simulink model "MicrogridControl"  (R2025b)
settings: Solver=VariableStepAuto  StartTime=0.0  StopTime=8  FixedStep=Ts  RelTol=1e-3
PreLoadFcn:
  | NormalOperation;
  | MicrogridControlParam;
undefined symbols (not defined in the file): base, bessModeInitial, bessSystem, bessVoltage, breakerStatus, DiscIntNeverNeededParam, ee_sli_rtmsupport, event, gcbh, generator, gflInverter, gfmInverter, Inertia, lineInductance, lineResistance, machine, plannedIsland, pmsm, powerLimit, powerQuality, PV, PVInverter, ref, resync, solar, solarInsolationChange, systemFrequency, Ts, windController, windSystem, windTurbine
libraries: nesl_utility x234, ee_lib x174, fl_lib x143, eeGeneralControl x137, simulink x78, eeTransforms x47, slpidlib x23, nesl_utility_internal x12, eePwmGenerator x9, eeSinusoidalMeasurementV2 x9, custom_lib x7, batteryecm_lib x6
(part 13 of 25)

== system MicrogridControl/BESS/BESS Integrated1/Detailed/BESS Plant/Converter ==
  mabc : Inport
  Average : Subsystem  VariantControl=Average
  Switching : Subsystem  VariantControl=Switching
  + : PMIOPort  Side=Left
  - : PMIOPort  Port=2  Side=Left
  ~ : PMIOPort  Port=3  Side=Right

== system MicrogridControl/BESS/BESS Integrated1/Detailed/Filter & Measurements/PLL & Measurements ==
  V : Inport
  I : Inport  Port=2
  Measurement1 : Subsystem
  Measurement2 : Subsystem
  Subsystem : Subsystem
  Out Bus Element : Outport  PortName=VIbus  Element=Vq
  Out Bus Element1 : Outport  PortName=VIbus  Element=Vd
  Out Bus Element2 : Outport  PortName=VIbus  Element=Freq
  Out Bus Element3 : Outport  PortName=VIbus  Element=Theta
  Out Bus Element4 : Outport  PortName=VIbus  Element=Vmag
  Out Bus Element5 : Outport  PortName=VIbus  Element=Iq
  Out Bus Element6 : Outport  PortName=VIbus  Element=Id
  Out Bus Element7 : Outport  PortName=VIbus  Element=Iabc
  Out Bus Element8 : Outport  PortName=VIbus  Element=Vabc
  wires:
  Subsystem/6(Id1) -> Out Bus Element6/1
  Subsystem/7(Iq1) -> Out Bus Element5/1
  Measurement1/1(Vg) -> Subsystem/2(Iabc), Out Bus Element7/1
  I/1 -> Measurement1/1(u)
  Subsystem/1(mag) -> Out Bus Element4/1
  Measurement2/1(Vg) -> Subsystem/1(Vabc), Out Bus Element8/1
  Subsystem/4(Vd) -> Out Bus Element1/1
  Subsystem/3(angle) -> Out Bus Element3/1
  Subsystem/5(Vq) -> Out Bus Element/1
  Subsystem/2(freq) -> Out Bus Element2/1
  V/1 -> Measurement2/1(u)

== system MicrogridControl/BESS/BESS Integrated1/Simplified/Grid Following/Measurements ==
  Current and Voltage Sensor (Three-Phase)5 : ee_lib/Sensors & Transducers/Current and Voltage Sensor (Three-Phase)  vMeasurementType=ee.enum.vmeasurement.lg  outputUnit=ee.enum.unit.pu  SRated=plantRating*1000 A*V  VRated=Vac V  I_specify=off  I_priority=None  I=[0, 0, 0] A  I_nominal_specify=off  I_nominal_value=1  I_nominal_unit=A  V_specify=off  V_priority=None  V=[0, 0, 0] V  V_nominal_specify=off  V_nominal_value=1  V_nominal_unit=V
      settings: InternalSimscapePortConfiguration="{\"Bottom\":[],\"Left\":[{\"id\":\"N1\",\"label\":\"~1\",\"type\":\"foundation.electrical.three_phase\"}],\"Right\":[{\"id\":\"V_output\",\"label\":\"V\",\"type\":\"output\"},{\"id\":\"I_output\",\"label\":\"I\",\"type\":\"output\"},{\"id\":\"N2\",\"label\":\"~2\",\"type\":\"foundation.electrical.three_phase\"}],\"Top\":[]}"
  Gain1 : Gain  Gain=1/(plantRating*1000)
  Gain2 : Gain  Gain=1/(plantRating*1000)
  Low-Pass Filter (Discrete or Continuous)1 : eeGeneralControl/Low-Pass Filter (Discrete or Continuous)  K=1  T=0.1  B=inf  A=-inf  init_option=Inherited from block input  x0=0  Ts=-1
  Low-Pass Filter (Discrete or Continuous)2 : eeGeneralControl/Low-Pass Filter (Discrete or Continuous)  K=1  T=0.1  B=inf  A=-inf  init_option=Inherited from block input  x0=0  Ts=-1
  PS-Simulink Converter{,1..3} (4 alike) : nesl_utility/PS-Simulink Converter  PhysicalDomain=network_engine_domain  SubClassName=ps_output  LeftPortType=input  RightPortType=output  PseudoPeriodic=off  Frequencies=[]  VectorFormat=inherit  Unit=inherit  AffineConversion=off
  Power Sensor (Three-Phase) : ee_lib/Sensors & Transducers/Power Sensor (Three-Phase)  load_type=ee.enum.passive.type_balanced.balanced  f0=60 Hz
      settings: InternalSimscapePortConfiguration="{\"Bottom\":[],\"Left\":[{\"id\":\"N1\",\"label\":\"~1\",\"type\":\"foundation.electrical.three_phase\"}],\"Right\":[{\"id\":\"N2\",\"label\":\"~2\",\"type\":\"foundation.electrical.three_phase\"}],\"Top\":[{\"id\":\"Pm\",\"label\":\"P\",\"type\":\"output\"},{\"id\":\"Qm\",\"label\":\"Q\",\"type\":\"output\"}]}"
  In : PMIOPort  Side=Left
  ~ : PMIOPort  Port=2  Side=Right
  P : Outport
  Q : Outport  Port=2
  V : Outport  Port=3
  I : Outport  Port=4
  wires:
  Gain2/1 -> Q/1
  Gain1/1 -> P/1
  PS-Simulink Converter3/1 -> I/1
  PS-Simulink Converter2/1 -> V/1
  Low-Pass Filter (Discrete or Continuous)2/1 -> Gain2/1
  Low-Pass Filter (Discrete or Continuous)1/1 -> Gain1/1
  PS-Simulink Converter1/1 -> Low-Pass Filter (Discrete or Continuous)2/1
  PS-Simulink Converter/1 -> Low-Pass Filter (Discrete or Continuous)1/1
  connections:
  PS-Simulink Converter3/LConn1 -- Current and Voltage Sensor (Three-Phase)5/RConn2
  Power Sensor (Three-Phase)/RConn1 -- Current and Voltage Sensor (Three-Phase)5/LConn1
  PS-Simulink Converter1/LConn1 -- Power Sensor (Three-Phase)/LConn3
  ~/RConn1 -- Current and Voltage Sensor (Three-Phase)5/RConn3
  In/RConn1 -- Power Sensor (Three-Phase)/LConn1
  PS-Simulink Converter/LConn1 -- Power Sensor (Three-Phase)/LConn2
  PS-Simulink Converter2/LConn1 -- Current and Voltage Sensor (Three-Phase)5/RConn1

== system MicrogridControl/BESS/BESS Integrated1/Simplified/Grid Following/Power Limiter ==
  P : Inport
  SOC : Inport  Port=2
  V : Inport  Port=3
  Add : Sum
  Compare To Constant : simulink/Logic and Bit Operations/Compare To Constant  relop=<=  const=minSOC  OutDataTypeStr=boolean
  Compare To Constant1 : simulink/Logic and Bit Operations/Compare To Constant  relop=>=  const=maxSOC  OutDataTypeStr=boolean
  Constant : Constant  Value=maxSOC
  Constant1 : Constant  Value=0
  Constant2 : Constant  Value=minSOC
  Constant3 : Constant  Value=0
  Constant5 : Constant  Value=minSOC
  Data Type Conversion : DataTypeConversion  OutDataTypeStr=double  SaturateOnIntegerOverflow=off  RndMeth=Floor
  Delay1 : Delay  DelayLength=1
  Divide : Product  Inputs=*/
  Gain : Gain  Gain=-1/(Inf)
  GreaterThan : RelationalOperator  Operator=>  OutDataTypeStr=boolean  RndMeth=Simplest  InputSameDT=off
  GreaterThan1 : RelationalOperator  Operator=<  OutDataTypeStr=boolean  RndMeth=Simplest  InputSameDT=off
  GreaterThan3 : RelationalOperator  Operator=<  OutDataTypeStr=boolean  RndMeth=Simplest  InputSameDT=off
  NOR : Logic  Operator=NOR  IconShape=distinctive  AllPortsSameDT=off  OutDataTypeStr=boolean
  Product : Product
  Scope1 : Scope  NumInputPorts=2
  Scope2 : Scope
  Scope3 : Scope  NumInputPorts=3
  Switch : Switch  Criteria=u2 > Threshold  SaturateOnIntegerOverflow=off  InputSameDT=off
  Switch1 : Switch  Criteria=u2 > Threshold  SaturateOnIntegerOverflow=off  InputSameDT=off
  Switch2 : Switch  Criteria=u2 > Threshold  SaturateOnIntegerOverflow=off  InputSameDT=off
  POut : Outport
  SOCFlag : Outport  Port=2
  wires:
  Product/1 -> POut/1
  Gain/1 -> Add/1
  Data Type Conversion/1 -> Product/2
  NOR/1 -> Data Type Conversion/1
  Compare To Constant1/1 -> NOR/2
  Compare To Constant/1 -> NOR/1
  Add/1 -> Compare To Constant1/1, Compare To Constant/1
  Switch2/1 -> Product/1, Divide/1
  Switch/1 -> Switch2/3, Scope3/3
  SOC/1 -> GreaterThan/1, GreaterThan1/1, Scope2/1, GreaterThan3/1, Add/2
  Divide/1 -> Gain/1
  Delay1/1 -> Divide/2
  V/1 -> Delay1/1
  GreaterThan3/1 -> SOCFlag/1
  Constant5/1 -> GreaterThan3/2
  Constant/1 -> GreaterThan/2
  GreaterThan/1 -> Switch/2
  Constant1/1 -> Switch/1
  Constant2/1 -> GreaterThan1/2
  GreaterThan1/1 -> Switch1/2, Scope1/1
  Constant3/1 -> Switch1/1
  Switch1/1 -> Switch2/1, Scope3/1
  P/1 -> Switch/3, Switch1/3, Switch2/2, Scope3/2

== system MicrogridControl/BESS/BESS Integrated1/Simplified/Grid Following/SOC Estimation ==
  I : Inport
  Constant : Constant  Value=0.95
  Gain : Gain  Gain=-1/(100000)
  Integrator (Discrete or Continuous) : eeGeneralControl/Integrator (Discrete or Continuous)  LabelModeActiveChoice=Discrete  IntegratorMethod=Integration: Forward Euler  ExternalReset=level  LimitType=Anti-windup  B=inf  A=-inf  Ts=-1
  SOC : Outport
  wires:
  Integrator (Discrete or Continuous)/1 -> SOC/1
  Gain/1 -> Integrator (Discrete or Continuous)/1
  I/1 -> Gain/1
  Constant/1 -> Integrator (Discrete or Continuous)/3

== system MicrogridControl/BESS/BESS Integrated1/Simplified/Grid Forming/Limiter ==
  SOC : Inport
  Compare To Constant : simulink/Logic and Bit Operations/Compare To Constant  relop=<=  const=minSOC  OutDataTypeStr=boolean
  Compare To Constant1 : simulink/Logic and Bit Operations/Compare To Constant  relop=>=  const=maxSOC  OutDataTypeStr=boolean
  Data Type Conversion : DataTypeConversion  OutDataTypeStr=double  SaturateOnIntegerOverflow=off  RndMeth=Floor
  Delay : Delay  DelayLength=1  InputProcessing=Columns as channels (frame based)
  OR : Logic  Operator=OR  AllPortsSameDT=off  OutDataTypeStr=boolean
  Flag : Outport
  wires:
  Delay/1 -> Flag/1
  Data Type Conversion/1 -> Delay/1
  OR/1 -> Data Type Conversion/1
  Compare To Constant1/1 -> OR/2
  Compare To Constant/1 -> OR/1
  SOC/1 -> Compare To Constant1/1, Compare To Constant/1

== system MicrogridControl/BESS/BESS Integrated1/Simplified/Grid Forming/Measurements ==
  Current and Voltage Sensor (Three-Phase)5 : ee_lib/Sensors & Transducers/Current and Voltage Sensor (Three-Phase)  vMeasurementType=ee.enum.vmeasurement.lg  outputUnit=ee.enum.unit.pu  SRated=plantRating*1000 A*V  VRated=Vac V  I_specify=off  I_priority=None  I=[0, 0, 0] A  I_nominal_specify=off  I_nominal_value=1  I_nominal_unit=A  V_specify=off  V_priority=None  V=[0, 0, 0] V  V_nominal_specify=off  V_nominal_value=1  V_nominal_unit=V
      settings: InternalSimscapePortConfiguration="{\"Bottom\":[],\"Left\":[{\"id\":\"N1\",\"label\":\"~1\",\"type\":\"foundation.electrical.three_phase\"}],\"Right\":[{\"id\":\"V_output\",\"label\":\"V\",\"type\":\"output\"},{\"id\":\"I_output\",\"label\":\"I\",\"type\":\"output\"},{\"id\":\"N2\",\"label\":\"~2\",\"type\":\"foundation.electrical.three_phase\"}],\"Top\":[]}"
  Gain1 : Gain  Gain=1/(plantRating*1000)
  Gain2 : Gain  Gain=1/(plantRating*1000)
  PS-Simulink Converter{,1..3} (4 alike) : nesl_utility/PS-Simulink Converter  PhysicalDomain=network_engine_domain  SubClassName=ps_output  LeftPortType=input  RightPortType=output  PseudoPeriodic=off  Frequencies=[]  VectorFormat=inherit  Unit=inherit  AffineConversion=off
  Power Sensor (Three-Phase) : ee_lib/Sensors & Transducers/Power Sensor (Three-Phase)  load_type=ee.enum.passive.type_balanced.balanced  f0=60 Hz
      settings: InternalSimscapePortConfiguration="{\"Bottom\":[],\"Left\":[{\"id\":\"N1\",\"label\":\"~1\",\"type\":\"foundation.electrical.three_phase\"}],\"Right\":[{\"id\":\"N2\",\"label\":\"~2\",\"type\":\"foundation.electrical.three_phase\"}],\"Top\":[{\"id\":\"Pm\",\"label\":\"P\",\"type\":\"output\"},{\"id\":\"Qm\",\"label\":\"Q\",\"type\":\"output\"}]}"
  In : PMIOPort  Side=Left
  ~ : PMIOPort  Port=2  Side=Right
  P : Outport
  Q : Outport  Port=2
  V : Outport  Port=3
  I : Outport  Port=4
  wires:
  PS-Simulink Converter1/1 -> Gain2/1
  PS-Simulink Converter/1 -> Gain1/1
  PS-Simulink Converter2/1 -> V/1
  PS-Simulink Converter3/1 -> I/1
  Gain1/1 -> P/1
  Gain2/1 -> Q/1
  connections:
  PS-Simulink Converter2/LConn1 -- Current and Voltage Sensor (Three-Phase)5/RConn1
  PS-Simulink Converter/LConn1 -- Power Sensor (Three-Phase)/LConn2
  In/RConn1 -- Power Sensor (Three-Phase)/LConn1
  ~/RConn1 -- Current and Voltage Sensor (Three-Phase)5/RConn3
  PS-Simulink Converter1/LConn1 -- Power Sensor (Three-Phase)/LConn3
  Power Sensor (Three-Phase)/RConn1 -- Current and Voltage Sensor (Three-Phase)5/LConn1
  PS-Simulink Converter3/LConn1 -- Current and Voltage Sensor (Three-Phase)5/RConn2

== system MicrogridControl/BESS/BESS Integrated1/Simplified/Grid Forming/Reference Generator ==
  Mode : Inport
  PRef : Inport  Port=2
  P : Inport  Port=3
  QRef : Inport  Port=4
  Q : Inport  Port=5
  VRef : Inport  Port=6
  V : Inport  Port=7
  Gain : Gain  Gain=efficiency/100
  Gain2 : Gain  Gain=sqrt(3)/Vac
  If : If
  If Action Subsystem : Subsystem  TreatAsAtomicUnit=on
  If Action Subsystem1 : Subsystem  TreatAsAtomicUnit=on
  Merge : Merge
  Merge1 : Merge
  Vt : Outport
  Ph : Outport  Port=2
  wires:
  Gain/1 -> If Action Subsystem/1(PRef)
  Mode/1 -> If/1
  If/1 -> If Action Subsystem/Action
  PRef/1 -> Gain/1, If Action Subsystem1/1(PRef)
  QRef/1 -> If Action Subsystem/3(QRef)
  VRef/1 -> If Action Subsystem1/3(VRef)
  V/1 -> Gain2/1
  If/2 -> If Action Subsystem1/Action
  If Action Subsystem/1(Vt) -> Merge/1
  If Action Subsystem1/1(Vt) -> Merge/2
  If Action Subsystem/2(Ph) -> Merge1/1
  If Action Subsystem1/2(Ph) -> Merge1/2
  Merge1/1 -> Ph/1
  P/1 -> If Action Subsystem/2(P), If Action Subsystem1/2(P)
  Q/1 -> If Action Subsystem/4(Q)
  Gain2/1 -> If Action Subsystem1/4(V)
  Merge/1 -> Vt/1

== system MicrogridControl/BESS/BESS Integrated1/Simplified/Grid Forming/SOC Estimation ==
  P : Inport
  Constant : Constant  Value=Vdc
  Constant1 : Constant  Value=initialSOC
  Constant2 : Constant  Value=capacity
  Constant3 : Constant  Value=Inf
  Divide : Product  Inputs=*/
  Divide1 : Product  Inputs=*/
  Gain : Gain  Gain=-plantRating*1000
  Integrator (Discrete or Continuous) : eeGeneralControl/Integrator (Discrete or Continuous)  LabelModeActiveChoice=Discrete  IntegratorMethod=Integration: Forward Euler  ExternalReset=level  LimitType=Anti-windup  B=inf  A=-inf  Ts=-1
  String Compare : StringCompare
  String Constant : StringConstant  String=capacityType
  String Constant1 : StringConstant  String="\"Fixed\""
  Switch : Switch  Criteria=u2 > Threshold  SaturateOnIntegerOverflow=off  InputSameDT=off
  Meas : Outport
  wires:
  Gain/1 -> Divide/1
  P/1 -> Gain/1
  Constant/1 -> Divide/2
  Divide/1 -> Divide1/1
  Constant1/1 -> Integrator (Discrete or Continuous)/3
  Integrator (Discrete or Continuous)/1 -> Meas/1
  String Constant/1 -> String Compare/1
  String Constant1/1 -> String Compare/2
  String Compare/1 -> Switch/2
  Switch/1 -> Divide1/2
  Divide1/1 -> Integrator (Discrete or Continuous)/1
  Constant2/1 -> Switch/1
  Constant3/1 -> Switch/3

== system MicrogridControl/BESS/BESS Integrated3/Detailed/BESS Controller/Grid Following ==
  VRef : Inport
  FRef : Inport  Port=2
  PRef : Inport  Port=3
  QRef : Inport  Port=4
  Mode : Inport  Port=5
  Reset : Inport  Port=6
  In Bus Element3 : Inport  Port=7  PortName=VIBus  Element=Vd
  BusElementIn : Inport  Port=7  PortName=VIBus  Element=Vd
  In Bus Element2 : Inport  Port=7  PortName=VIBus  Element=Vq
  In Bus Element7 : Inport  Port=7  PortName=VIBus  Element=Theta
  BusElementIn1 : Inport  Port=7  PortName=VIBus  Element=Freq
  BusElementIn3 : Inport  Port=7  PortName=VIBus  Element=Id
  BusElementIn4 : Inport  Port=7  PortName=VIBus  Element=Iq
  Constant : Constant  Value=10
  Current_controller : Subsystem
  Inverse Park Transform1 : eeTransforms/Inverse Park Transform  AxisAlignment=Q-axis  PowerInvariant=off
  Reference Current : Subsystem
  Sum2 : Sum  Inputs=|+-
  Terminator : Terminator
  Terminator1 : Terminator
  Unit Delay : UnitDelay  SampleTime=Td  HasFrameUpgradeWarning=on
  Unit Delay1 : UnitDelay  SampleTime=Td  HasFrameUpgradeWarning=on
  Unit Delay2 : UnitDelay  SampleTime=Ts  HasFrameUpgradeWarning=on
  mabc : Outport
  wires:
  QRef/1 -> Reference Current/6(QRef)
  PRef/1 -> Reference Current/5(PRef)
  BusElementIn4/1 -> Current_controller/4(iq)
  BusElementIn3/1 -> Current_controller/2(ipvd)
  BusElementIn1/1 -> Unit Delay1/1
  BusElementIn/1 -> Unit Delay/1
  Unit Delay/1 -> Reference Current/2(V-mag)
  Unit Delay1/1 -> Sum2/2
  Reference Current/1(id_ref) -> Current_controller/1(id-ref)
  Reference Current/2(iq_ref) -> Current_controller/3(iqref)
  Sum2/1 -> Reference Current/3(del f)
  VRef/1 -> Reference Current/1(V_ref)
  FRef/1 -> Sum2/1
  In Bus Element7/1 -> Inverse Park Transform1/2
  In Bus Element3/1 -> Current_controller/5(Vd)
  Current_controller/1(mdq0) -> Inverse Park Transform1/1
  Unit Delay2/1 -> mabc/1
  Inverse Park Transform1/1 -> Unit Delay2/1
  In Bus Element2/1 -> Current_controller/6(Vq)
  Mode/1 -> Terminator/1
  Reset/1 -> Terminator1/1
  Constant/1 -> Reference Current/4(LVRT_iq)

== system MicrogridControl/BESS/BESS Integrated3/Detailed/BESS Controller/Grid Forming ==
  VRef : Inport
  FRef : Inport  Port=2
  PRef : Inport  Port=3
  QRef : Inport  Port=4
  Mode : Inport  Port=5
  Reset : Inport  Port=6
  Bus Element In : Inport  Port=7  PortName=VIBus  Element=Vabc
  BusElementIn : Inport  Port=7  PortName=VIBus  Element=Iabc
  Current Limiting : Subsystem
  Grid Voltage Reactive Power Support : Subsystem
  Measurement : Subsystem
      mask Display: image('meas2_1_7_7_2_2.png');
  Power Control : Subsystem
  Subsystem2 : Subsystem
      settings: PortSchema="{\"entries\":[{\"content\":{\"sides\":[{\"content\":{\"connectorIds\":[\"Out1\"]},\"type\":\"ConnectorPlacement.EquallySpacedRectSide\",\"uuid\":\"7526c1f7-0aba-4355-8bbd-47d168879ecb\"},{\"content\":{\"connectorIds\":[\"In1\",\"In2\"],\"side\":\"RIGHT\"},\"type\":\"ConnectorPlacement.EquallySpacedRectSide\",\"uuid\":\"1dda9693-ec76-4df0-8ad4-aaa83d2574b3\"},{\"content\":{\"side\":\"TOP\"},\"type\":\"ConnectorPlacement.EquallySpacedRectSide\",\"uuid\":\"71ea411b-eb5f-4279-ae23-08ebb3ff1ed6\"}]},\"type\":\"ConnectorPlacement.EquallySpacedConnector\",\"uuid\":\"19864e0c-0998-460d-9705-13c69283d4ec\"}],\"packageUris\":[\"http://schema.mathworks.com/mf0/Connector/R2020b\"],\"version\":\"1.0\"}"
  Terminator : Terminator
  Terminator1 : Terminator
  Terminator2 : Terminator
  VoltageCurrentControl : Subsystem
      settings: PortSchema="{\"entries\":[{\"content\":{\"sides\":[{\"content\":{\"connectorIds\":[\"In1\",\"In2\",\"In3\"]},\"type\":\"ConnectorPlacement.EquallySpacedRectSide\",\"uuid\":\"0bf15a12-7bc0-47e4-89bd-435769673763\"},{\"content\":{\"connectorIds\":[\"Out1\"],\"side\":\"RIGHT\"},\"type\":\"ConnectorPlacement.EquallySpacedRectSide\",\"uuid\":\"44a15d74-8878-4ec6-abe4-be0b1b609519\"},{\"content\":{\"connectorIds\":[\"In4\"],\"side\":\"TOP\"},\"type\":\"ConnectorPlacement.EquallySpacedRectSide\",\"uuid\":\"7a96781e-5638-4b2a-8101-d5785aae9f0f\"}]},\"type\":\"ConnectorPlacement.EquallySpacedConnector\",\"uuid\":\"4b3373ad-cf20-4175-894e-3bd1604dd0ce\"}],\"packageUris\":[\"http://schema.mathworks.com/mf0/Connector/R2020b\"],\"version\":\"1.0\"}"
  mabc : Outport
  wires:
  Reset/1 -> Subsystem2/2(Reset), VoltageCurrentControl/3(Reset)
  Mode/1 -> Power Control/6(CntrlFlag)
  VRef/1 -> Power Control/4(Vref)
  FRef/1 -> Power Control/5(Fref)
  Measurement/4(fmeas) -> Terminator2/1
  Grid Voltage Reactive Power Support/2(Qref) -> Power Control/3(Qref)
  Grid Voltage Reactive Power Support/1(Pref) -> Power Control/2(Pref)
  PRef/1 -> Grid Voltage Reactive Power Support/2(PrefInput)
  QRef/1 -> Grid Voltage Reactive Power Support/3(QrefInput)
  Current Limiting/1(currentLimiting) -> VoltageCurrentControl/1(currentLimiting)
  Power Control/2(activeControl) -> VoltageCurrentControl/2(activeControl)
  Power Control/1(reactiveControl) -> Current Limiting/2(reactiveControl)
  Power Control/3(angle) -> Measurement/3(Angle)
  Measurement/1(measure) -> Grid Voltage Reactive Power Support/1(measure), Power Control/1(measure), VoltageCurrentControl/4(measure), Current Limiting/1(measure)
  Measurement/3(Qmeas) -> Terminator1/1
  Measurement/2(Pmeas) -> Terminator/1
  BusElementIn/1 -> Measurement/2(Igabc)
  Bus Element In/1 -> Measurement/1(Vgabcc)
  VoltageCurrentControl/1(mabc) -> Subsystem2/1(In)
  Subsystem2/1(mabc) -> mabc/1

== system MicrogridControl/BESS/BESS Integrated3/Detailed/BESS Plant/Converter ==
  mabc : Inport
  Average : Subsystem  VariantControl=Average
  Switching : Subsystem  VariantControl=Switching
  + : PMIOPort  Side=Left
  - : PMIOPort  Port=2  Side=Left
  ~ : PMIOPort  Port=3  Side=Right

== system MicrogridControl/BESS/BESS Integrated3/Detailed/Filter & Measurements/PLL & Measurements ==
  V : Inport
  I : Inport  Port=2
  Measurement1 : Subsystem
  Measurement2 : Subsystem
  Subsystem : Subsystem
  Out Bus Element : Outport  PortName=VIbus  Element=Vq
  Out Bus Element1 : Outport  PortName=VIbus  Element=Vd
  Out Bus Element2 : Outport  PortName=VIbus  Element=Freq
  Out Bus Element3 : Outport  PortName=VIbus  Element=Theta
  Out Bus Element4 : Outport  PortName=VIbus  Element=Vmag
  Out Bus Element5 : Outport  PortName=VIbus  Element=Iq
  Out Bus Element6 : Outport  PortName=VIbus  Element=Id
  Out Bus Element7 : Outport  PortName=VIbus  Element=Iabc
  Out Bus Element8 : Outport  PortName=VIbus  Element=Vabc
  wires:
  Subsystem/6(Id1) -> Out Bus Element6/1
  Subsystem/7(Iq1) -> Out Bus Element5/1
  Measurement1/1(Vg) -> Subsystem/2(Iabc), Out Bus Element7/1
  I/1 -> Measurement1/1(u)
  Subsystem/1(mag) -> Out Bus Element4/1
  Measurement2/1(Vg) -> Subsystem/1(Vabc), Out Bus Element8/1
  Subsystem/4(Vd) -> Out Bus Element1/1
  Subsystem/3(angle) -> Out Bus Element3/1
  Subsystem/5(Vq) -> Out Bus Element/1
  Subsystem/2(freq) -> Out Bus Element2/1
  V/1 -> Measurement2/1(u)

== system MicrogridControl/BESS/BESS Integrated3/Simplified/Grid Following/Measurements ==
  Current and Voltage Sensor (Three-Phase)5 : ee_lib/Sensors & Transducers/Current and Voltage Sensor (Three-Phase)  vMeasurementType=ee.enum.vmeasurement.lg  outputUnit=ee.enum.unit.pu  SRated=plantRating*1000 A*V  VRated=Vac V  I_specify=off  I_priority=None  I=[0, 0, 0] A  I_nominal_specify=off  I_nominal_value=1  I_nominal_unit=A  V_specify=off  V_priority=None  V=[0, 0, 0] V  V_nominal_specify=off  V_nominal_value=1  V_nominal_unit=V
      settings: InternalSimscapePortConfiguration="{\"Bottom\":[],\"Left\":[{\"id\":\"N1\",\"label\":\"~1\",\"type\":\"foundation.electrical.three_phase\"}],\"Right\":[{\"id\":\"V_output\",\"label\":\"V\",\"type\":\"output\"},{\"id\":\"I_output\",\"label\":\"I\",\"type\":\"output\"},{\"id\":\"N2\",\"label\":\"~2\",\"type\":\"foundation.electrical.three_phase\"}],\"Top\":[]}"
  Gain1 : Gain  Gain=1/(plantRating*1000)
  Gain2 : Gain  Gain=1/(plantRating*1000)
  Low-Pass Filter (Discrete or Continuous)1 : eeGeneralControl/Low-Pass Filter (Discrete or Continuous)  K=1  T=0.1  B=inf  A=-inf  init_option=Inherited from block input  x0=0  Ts=-1
  Low-Pass Filter (Discrete or Continuous)2 : eeGeneralControl/Low-Pass Filter (Discrete or Continuous)  K=1  T=0.1  B=inf  A=-inf  init_option=Inherited from block input  x0=0  Ts=-1
  PS-Simulink Converter{,1..3} (4 alike) : nesl_utility/PS-Simulink Converter  PhysicalDomain=network_engine_domain  SubClassName=ps_output  LeftPortType=input  RightPortType=output  PseudoPeriodic=off  Frequencies=[]  VectorFormat=inherit  Unit=inherit  AffineConversion=off
  Power Sensor (Three-Phase) : ee_lib/Sensors & Transducers/Power Sensor (Three-Phase)  load_type=ee.enum.passive.type_balanced.balanced  f0=60 Hz
      settings: InternalSimscapePortConfiguration="{\"Bottom\":[],\"Left\":[{\"id\":\"N1\",\"label\":\"~1\",\"type\":\"foundation.electrical.three_phase\"}],\"Right\":[{\"id\":\"N2\",\"label\":\"~2\",\"type\":\"foundation.electrical.three_phase\"}],\"Top\":[{\"id\":\"Pm\",\"label\":\"P\",\"type\":\"output\"},{\"id\":\"Qm\",\"label\":\"Q\",\"type\":\"output\"}]}"
  In : PMIOPort  Side=Left
  ~ : PMIOPort  Port=2  Side=Right
  P : Outport
  Q : Outport  Port=2
  V : Outport  Port=3
  I : Outport  Port=4
  wires:
  Gain2/1 -> Q/1
  Gain1/1 -> P/1
  PS-Simulink Converter3/1 -> I/1
  PS-Simulink Converter2/1 -> V/1
  Low-Pass Filter (Discrete or Continuous)2/1 -> Gain2/1
  Low-Pass Filter (Discrete or Continuous)1/1 -> Gain1/1
  PS-Simulink Converter1/1 -> Low-Pass Filter (Discrete or Continuous)2/1
  PS-Simulink Converter/1 -> Low-Pass Filter (Discrete or Continuous)1/1
  connections:
  PS-Simulink Converter3/LConn1 -- Current and Voltage Sensor (Three-Phase)5/RConn2
  Power Sensor (Three-Phase)/RConn1 -- Current and Voltage Sensor (Three-Phase)5/LConn1
  PS-Simulink Converter1/LConn1 -- Power Sensor (Three-Phase)/LConn3
  ~/RConn1 -- Current and Voltage Sensor (Three-Phase)5/RConn3
  In/RConn1 -- Power Sensor (Three-Phase)/LConn1
  PS-Simulink Converter/LConn1 -- Power Sensor (Three-Phase)/LConn2
  PS-Simulink Converter2/LConn1 -- Current and Voltage Sensor (Three-Phase)5/RConn1

== system MicrogridControl/BESS/BESS Integrated3/Simplified/Grid Following/Power Limiter ==
  P : Inport
  SOC : Inport  Port=2
  V : Inport  Port=3
  Add : Sum
  Compare To Constant : simulink/Logic and Bit Operations/Compare To Constant  relop=<=  const=minSOC  OutDataTypeStr=boolean
  Compare To Constant1 : simulink/Logic and Bit Operations/Compare To Constant  relop=>=  const=maxSOC  OutDataTypeStr=boolean
  Constant : Constant  Value=maxSOC
  Constant1 : Constant  Value=0
  Constant2 : Constant  Value=minSOC
  Constant3 : Constant  Value=0
  Constant5 : Constant  Value=minSOC
  Data Type Conversion : DataTypeConversion  OutDataTypeStr=double  SaturateOnIntegerOverflow=off  RndMeth=Floor
  Delay1 : Delay  DelayLength=1
  Divide : Product  Inputs=*/
  Gain : Gain  Gain=-1/(Inf)
  GreaterThan : RelationalOperator  Operator=>  OutDataTypeStr=boolean  RndMeth=Simplest  InputSameDT=off
  GreaterThan1 : RelationalOperator  Operator=<  OutDataTypeStr=boolean  RndMeth=Simplest  InputSameDT=off
  GreaterThan3 : RelationalOperator  Operator=<  OutDataTypeStr=boolean  RndMeth=Simplest  InputSameDT=off
  NOR : Logic  Operator=NOR  IconShape=distinctive  AllPortsSameDT=off  OutDataTypeStr=boolean
  Product : Product
  Scope1 : Scope  NumInputPorts=2
  Scope2 : Scope
  Scope3 : Scope  NumInputPorts=3
  Switch : Switch  Criteria=u2 > Threshold  SaturateOnIntegerOverflow=off  InputSameDT=off
  Switch1 : Switch  Criteria=u2 > Threshold  SaturateOnIntegerOverflow=off  InputSameDT=off
  Switch2 : Switch  Criteria=u2 > Threshold  SaturateOnIntegerOverflow=off  InputSameDT=off
  POut : Outport
  SOCFlag : Outport  Port=2
  wires:
  Product/1 -> POut/1
  Gain/1 -> Add/1
  Data Type Conversion/1 -> Product/2
  NOR/1 -> Data Type Conversion/1
  Compare To Constant1/1 -> NOR/2
  Compare To Constant/1 -> NOR/1
  Add/1 -> Compare To Constant1/1, Compare To Constant/1
  Switch2/1 -> Product/1, Divide/1
  Switch/1 -> Switch2/3, Scope3/3
  SOC/1 -> GreaterThan/1, GreaterThan1/1, Scope2/1, GreaterThan3/1, Add/2
  Divide/1 -> Gain/1
  Delay1/1 -> Divide/2
  V/1 -> Delay1/1
  GreaterThan3/1 -> SOCFlag/1
  Constant5/1 -> GreaterThan3/2
  Constant/1 -> GreaterThan/2
  GreaterThan/1 -> Switch/2
  Constant1/1 -> Switch/1
  Constant2/1 -> GreaterThan1/2
  GreaterThan1/1 -> Switch1/2, Scope1/1
  Constant3/1 -> Switch1/1
  Switch1/1 -> Switch2/1, Scope3/1
  P/1 -> Switch/3, Switch1/3, Switch2/2, Scope3/2

== system MicrogridControl/BESS/BESS Integrated3/Simplified/Grid Following/SOC Estimation ==
  I : Inport
  Constant : Constant  Value=0.95
  Gain : Gain  Gain=-1/(100000)
  Integrator (Discrete or Continuous) : eeGeneralControl/Integrator (Discrete or Continuous)  LabelModeActiveChoice=Discrete  IntegratorMethod=Integration: Forward Euler  ExternalReset=level  LimitType=Anti-windup  B=inf  A=-inf  Ts=-1
  SOC : Outport
  wires:
  Integrator (Discrete or Continuous)/1 -> SOC/1
  Gain/1 -> Integrator (Discrete or Continuous)/1
  I/1 -> Gain/1
  Constant/1 -> Integrator (Discrete or Continuous)/3

== system MicrogridControl/BESS/BESS Integrated3/Simplified/Grid Forming/Limiter ==
  SOC : Inport
  Compare To Constant : simulink/Logic and Bit Operations/Compare To Constant  relop=<=  const=minSOC  OutDataTypeStr=boolean
  Compare To Constant1 : simulink/Logic and Bit Operations/Compare To Constant  relop=>=  const=maxSOC  OutDataTypeStr=boolean
  Data Type Conversion : DataTypeConversion  OutDataTypeStr=double  SaturateOnIntegerOverflow=off  RndMeth=Floor
  Delay : Delay  DelayLength=1  InputProcessing=Columns as channels (frame based)
  OR : Logic  Operator=OR  AllPortsSameDT=off  OutDataTypeStr=boolean
  Flag : Outport
  wires:
  Delay/1 -> Flag/1
  Data Type Conversion/1 -> Delay/1
  OR/1 -> Data Type Conversion/1
  Compare To Constant1/1 -> OR/2
  Compare To Constant/1 -> OR/1
  SOC/1 -> Compare To Constant1/1, Compare To Constant/1

== system MicrogridControl/BESS/BESS Integrated3/Simplified/Grid Forming/Measurements ==
  Current and Voltage Sensor (Three-Phase)5 : ee_lib/Sensors & Transducers/Current and Voltage Sensor (Three-Phase)  vMeasurementType=ee.enum.vmeasurement.lg  outputUnit=ee.enum.unit.pu  SRated=plantRating*1000 A*V  VRated=Vac V  I_specify=off  I_priority=None  I=[0, 0, 0] A  I_nominal_specify=off  I_nominal_value=1  I_nominal_unit=A  V_specify=off  V_priority=None  V=[0, 0, 0] V  V_nominal_specify=off  V_nominal_value=1  V_nominal_unit=V
      settings: InternalSimscapePortConfiguration="{\"Bottom\":[],\"Left\":[{\"id\":\"N1\",\"label\":\"~1\",\"type\":\"foundation.electrical.three_phase\"}],\"Right\":[{\"id\":\"V_output\",\"label\":\"V\",\"type\":\"output\"},{\"id\":\"I_output\",\"label\":\"I\",\"type\":\"output\"},{\"id\":\"N2\",\"label\":\"~2\",\"type\":\"foundation.electrical.three_phase\"}],\"Top\":[]}"
  Gain1 : Gain  Gain=1/(plantRating*1000)
  Gain2 : Gain  Gain=1/(plantRating*1000)
  PS-Simulink Converter{,1..3} (4 alike) : nesl_utility/PS-Simulink Converter  PhysicalDomain=network_engine_domain  SubClassName=ps_output  LeftPortType=input  RightPortType=output  PseudoPeriodic=off  Frequencies=[]  VectorFormat=inherit  Unit=inherit  AffineConversion=off
  Power Sensor (Three-Phase) : ee_lib/Sensors & Transducers/Power Sensor (Three-Phase)  load_type=ee.enum.passive.type_balanced.balanced  f0=60 Hz
      settings: InternalSimscapePortConfiguration="{\"Bottom\":[],\"Left\":[{\"id\":\"N1\",\"label\":\"~1\",\"type\":\"foundation.electrical.three_phase\"}],\"Right\":[{\"id\":\"N2\",\"label\":\"~2\",\"type\":\"foundation.electrical.three_phase\"}],\"Top\":[{\"id\":\"Pm\",\"label\":\"P\",\"type\":\"output\"},{\"id\":\"Qm\",\"label\":\"Q\",\"type\":\"output\"}]}"
  In : PMIOPort  Side=Left
  ~ : PMIOPort  Port=2  Side=Right
  P : Outport
  Q : Outport  Port=2
  V : Outport  Port=3
  I : Outport  Port=4
  wires:
  PS-Simulink Converter1/1 -> Gain2/1
  PS-Simulink Converter/1 -> Gain1/1
  PS-Simulink Converter2/1 -> V/1
  PS-Simulink Converter3/1 -> I/1
  Gain1/1 -> P/1
  Gain2/1 -> Q/1
  connections:
  PS-Simulink Converter2/LConn1 -- Current and Voltage Sensor (Three-Phase)5/RConn1
  PS-Simulink Converter/LConn1 -- Power Sensor (Three-Phase)/LConn2
  In/RConn1 -- Power Sensor (Three-Phase)/LConn1
  ~/RConn1 -- Current and Voltage Sensor (Three-Phase)5/RConn3
  PS-Simulink Converter1/LConn1 -- Power Sensor (Three-Phase)/LConn3
  Power Sensor (Three-Phase)/RConn1 -- Current and Voltage Sensor (Three-Phase)5/LConn1
  PS-Simulink Converter3/LConn1 -- Current and Voltage Sensor (Three-Phase)5/RConn2

== system MicrogridControl/BESS/BESS Integrated3/Simplified/Grid Forming/Reference Generator ==
  Mode : Inport
  PRef : Inport  Port=2
  P : Inport  Port=3
  QRef : Inport  Port=4
  Q : Inport  Port=5
  VRef : Inport  Port=6
  V : Inport  Port=7
  Gain : Gain  Gain=efficiency/100
  Gain2 : Gain  Gain=sqrt(3)/Vac
  If : If
  If Action Subsystem : Subsystem  TreatAsAtomicUnit=on
  If Action Subsystem1 : Subsystem  TreatAsAtomicUnit=on
  Merge : Merge
  Merge1 : Merge
  Vt : Outport
  Ph : Outport  Port=2
  wires:
  Gain/1 -> If Action Subsystem/1(PRef)
  Mode/1 -> If/1
  If/1 -> If Action Subsystem/Action
  PRef/1 -> Gain/1, If Action Subsystem1/1(PRef)
  QRef/1 -> If Action Subsystem/3(QRef)
  VRef/1 -> If Action Subsystem1/3(VRef)
  V/1 -> Gain2/1
  If/2 -> If Action Subsystem1/Action
  If Action Subsystem/1(Vt) -> Merge/1
  If Action Subsystem1/1(Vt) -> Merge/2
  If Action Subsystem/2(Ph) -> Merge1/1
  If Action Subsystem1/2(Ph) -> Merge1/2
  Merge1/1 -> Ph/1
  P/1 -> If Action Subsystem/2(P), If Action Subsystem1/2(P)
  Q/1 -> If Action Subsystem/4(Q)
  Gain2/1 -> If Action Subsystem1/4(V)
  Merge/1 -> Vt/1

== system MicrogridControl/BESS/BESS Integrated3/Simplified/Grid Forming/SOC Estimation ==
  P : Inport
  Constant : Constant  Value=Vdc
  Constant1 : Constant  Value=initialSOC
  Constant2 : Constant  Value=capacity
  Constant3 : Constant  Value=Inf
  Divide : Product  Inputs=*/
  Divide1 : Product  Inputs=*/
  Gain : Gain  Gain=-plantRating*1000
  Integrator (Discrete or Continuous) : eeGeneralControl/Integrator (Discrete or Continuous)  LabelModeActiveChoice=Discrete  IntegratorMethod=Integration: Forward Euler  ExternalReset=level  LimitType=Anti-windup  B=inf  A=-inf  Ts=-1
  String Compare : StringCompare
  String Constant : StringConstant  String=capacityType
  String Constant1 : StringConstant  String="\"Fixed\""
  Switch : Switch  Criteria=u2 > Threshold  SaturateOnIntegerOverflow=off  InputSameDT=off
  Meas : Outport
  wires:
  Gain/1 -> Divide/1
  P/1 -> Gain/1
  Constant/1 -> Divide/2
  Divide/1 -> Divide1/1
  Constant1/1 -> Integrator (Discrete or Continuous)/3
  Integrator (Discrete or Continuous)/1 -> Meas/1
  String Constant/1 -> String Compare/1
  String Constant1/1 -> String Compare/2
  String Compare/1 -> Switch/2
  Switch/1 -> Divide1/2
  Divide1/1 -> Integrator (Discrete or Continuous)/1
  Constant2/1 -> Switch/1
  Constant3/1 -> Switch/3

== system MicrogridControl/Generator/Generator Integrated/Detailed/Governor and Prime Mover /Governor ==
  pu_velocity : Inport
  PRef : Inport  Port=2
  1/T_G : Gain  Gain=1/T_G
  1/droop : Gain  Gain=1/(droop_percentage/100)
  Delta load setpoint : Sum  Inputs=+-|
  Delta speed : Sum  Inputs=-+|
  Discrete-Time Integrator1 : DiscreteIntegrator  InitialCondition=pu_torque0  SampleTime=-1  ICPrevOutput=DiscIntNeverNeededParam  ICPrevScaledInput=DiscIntNeverNeededParam
  Scope : Scope  NumInputPorts=2
  Scope1 : Scope  NumInputPorts=2
  Speed_ref : Constant  Value=pu_speed_reference
  Subtract : Sum  Inputs=|+-
  delta_y : Outport  VectorParamsAs1DForOutWhenUnconnected=off
  wires:
  PRef/1 -> Delta load setpoint/1
  Discrete-Time Integrator1/1 -> Subtract/2, delta_y/1, Scope1/2
  1/T_G/1 -> Discrete-Time Integrator1/1
  Subtract/1 -> 1/T_G/1, Scope1/1
  Delta load setpoint/1 -> Subtract/1
  1/droop/1 -> Delta load setpoint/2
  pu_velocity/1 -> Delta speed/2, Scope/2
  Delta speed/1 -> 1/droop/1, Scope/1
  Speed_ref/1 -> Delta speed/1

== system MicrogridControl/Generator/Generator Integrated/Detailed/Governor and Prime Mover /Non-reheat turbine ==
  delta_y : Inport
  1/T_CH : Gain  Gain=1/T_CH
  Discrete-Time Integrator1 : DiscreteIntegrator  InitialCondition=pu_torque0  SampleTime=-1  ICPrevOutput=DiscIntNeverNeededParam  ICPrevScaledInput=DiscIntNeverNeededParam
  Scope : Scope  NumInputPorts=2
  Sum : Sum  Inputs=|+-
  torque : Outport  VectorParamsAs1DForOutWhenUnconnected=off
  wires:
  Discrete-Time Integrator1/1 -> torque/1, Scope/1, Sum/2
  1/T_CH/1 -> Discrete-Time Integrator1/1
  Sum/1 -> 1/T_CH/1
  delta_y/1 -> Sum/1, Scope/2

== system MicrogridControl/Microgrid Controller/Microgrid Control Functions/Black Start/Voltage Reference/Voltage Level 1 ==
  Enable : Inport
  Constant : Constant
  Constant1 : Constant  Value=0
  Constant2 : Constant  DisableCoverage=on  Value=-(delayLevel1)  OutDataTypeStr=Inherit: Inherit via back propagation  SampleTime=Ts
  Discrete-Time Integrator : DiscreteIntegrator  SampleTime=Ts  OutDataTypeStr=double  ICPrevOutput=DiscIntNeverNeededParam  ICPrevScaledInput=DiscIntNeverNeededParam
  Output : Sum  Inputs=|++  InputSameDT=on  SaturateOnIntegerOverflow=on  OutDataTypeStr=Inherit: Same as first input
  Product : Product  DisableCoverage=on  InputSameDT=on  SaturateOnIntegerOverflow=on  OutDataTypeStr=Inherit: Same as first input
  Saturation : Saturate  UpperLimit=voltageLevel1  LowerLimit=0
  Step : Step  Commented=on  DisableCoverage=on  Time=controllerBlackStart+delayLevel1  OutDataTypeStr=fixdt('double', 'DataTypeOverride', 'Off')  SampleTime=Ts
  Level 1 : Outport
  wires:
  Constant1/1 -> Output/2
  Constant/1 -> Product/1
  Enable/1 -> Discrete-Time Integrator/1
  Output/1 -> Saturation/1
  Product/1 -> Output/1
  Saturation/1 -> Level 1/1
  Discrete-Time Integrator/1 -> Product/2

== system MicrogridControl/Microgrid Controller/Microgrid Control Functions/Black Start/Voltage Reference/Voltage Level 2 ==
  Enable : Inport
  Constant : Constant
  Constant1 : Constant  Value=0
  Constant2 : Constant  Commented=on  DisableCoverage=on  Value=-(delayLevel2)  OutDataTypeStr=Inherit: Inherit via back propagation  SampleTime=Ts
  Discrete-Time Integrator : DiscreteIntegrator  SampleTime=Ts  OutDataTypeStr=double  ICPrevOutput=DiscIntNeverNeededParam  ICPrevScaledInput=DiscIntNeverNeededParam
  Output : Sum  Inputs=|++  InputSameDT=on  SaturateOnIntegerOverflow=on  OutDataTypeStr=Inherit: Same as first input
  Product : Product  DisableCoverage=on  InputSameDT=on  SaturateOnIntegerOverflow=on  OutDataTypeStr=Inherit: Same as first input
  Saturation : Saturate  UpperLimit=voltageLevel2  LowerLimit=0
  Step : Step  Commented=on  DisableCoverage=on  Time=delayLevel1+delayLevel2  OutDataTypeStr=fixdt('double', 'DataTypeOverride', 'Off')  SampleTime=Ts
  Level 2 : Outport
  wires:
  Constant1/1 -> Output/2
  Constant/1 -> Product/1
  Enable/1 -> Discrete-Time Integrator/1
  Discrete-Time Integrator/1 -> Product/2
  Saturation/1 -> Level 2/1
  Product/1 -> Output/1
  Output/1 -> Saturation/1

== system MicrogridControl/Microgrid Controller/Microgrid Control Functions/Black Start/Voltage Reference/Voltage Level 3 ==
  Enable : Inport
  Constant : Constant
  Constant1 : Constant  Value=0
  Constant2 : Constant  Commented=on  DisableCoverage=on  Value=-(delayLevel3+delayLevel3)  OutDataTypeStr=Inherit: Inherit via back propagation  SampleTime=Ts
  Discrete-Time Integrator : DiscreteIntegrator  SampleTime=Ts  OutDataTypeStr=double  ICPrevOutput=DiscIntNeverNeededParam  ICPrevScaledInput=DiscIntNeverNeededParam
  Output : Sum  Inputs=|++  InputSameDT=on  SaturateOnIntegerOverflow=on  OutDataTypeStr=Inherit: Same as first input
  Product : Product  DisableCoverage=on  InputSameDT=on  SaturateOnIntegerOverflow=on  OutDataTypeStr=Inherit: Same as first input
  Saturation : Saturate  UpperLimit=voltageLevel3  LowerLimit=0
  Step : Step  Commented=on  DisableCoverage=on  Time=delayLevel1+delayLevel2+delayLevel3  OutDataTypeStr=fixdt('double', 'DataTypeOverride', 'Off')  SampleTime=Ts
  Level 3 : Outport
  wires:
  Constant1/1 -> Output/2
  Constant/1 -> Product/1
  Enable/1 -> Discrete-Time Integrator/1
  Output/1 -> Saturation/1
  Product/1 -> Output/1
  Saturation/1 -> Level 3/1
  Discrete-Time Integrator/1 -> Product/2

== system MicrogridControl/Microgrid Controller/Microgrid Control Functions/Resynchronization/Synch Voltage/Subsystem2 ==
  MicrogridController : Inport
  ControlRoom : Inport  Port=2
  Constant : Constant  Value=1.05
  Switch : Switch  Criteria=u2 > Threshold  Threshold=0.5  SaturateOnIntegerOverflow=off  InputSameDT=off
  Out1 : Outport
  wires:
  MicrogridController/1 -> Switch/1
  ControlRoom/1 -> Switch/2
  Constant/1 -> Switch/3
  Switch/1 -> Out1/1

== system MicrogridControl/Microgrid Controller/Subsystem1/PLL/Frequency Measurement/Frequency Measurement ==
  abc : Inport
  Constant : Constant
  Discrete-Time Integrator : DiscreteIntegrator  SampleTime=sampleTime  LimitOutput=on  ICPrevOutput=DiscIntNeverNeededParam  ICPrevScaledInput=DiscIntNeverNeededParam
  If : If  IfExpression=u1 > 0.9
  If Action Subsystem : Subsystem  TreatAsAtomicUnit=on
  If Action Subsystem1 : Subsystem  TreatAsAtomicUnit=on
  Merge : Merge
  Postive Sequence : Subsystem
  Freq : Outport
  wires:
  Postive Sequence/1(posSeq) -> If Action Subsystem/1(V)
  Merge/1 -> Freq/1
  If Action Subsystem1/1(Out1) -> Merge/2
  If Action Subsystem/1(Freq) -> Merge/1
  Constant/1 -> Discrete-Time Integrator/1
  abc/1 -> Postive Sequence/1(abc)
  Discrete-Time Integrator/1 -> If/1, If Action Subsystem/2(Time)
  If/2 -> If Action Subsystem1/Action
  If/1 -> If Action Subsystem/Action

== system MicrogridControl/Microgrid Controller/Subsystem1/PLL1/Frequency Measurement/Frequency Measurement ==
  abc : Inport
  Constant : Constant
  Discrete-Time Integrator : DiscreteIntegrator  SampleTime=sampleTime  LimitOutput=on  ICPrevOutput=DiscIntNeverNeededParam  ICPrevScaledInput=DiscIntNeverNeededParam
  If : If  IfExpression=u1 > 0.9
  If Action Subsystem : Subsystem  TreatAsAtomicUnit=on
  If Action Subsystem1 : Subsystem  TreatAsAtomicUnit=on
  Merge : Merge
  Postive Sequence : Subsystem
  Freq : Outport
  wires:
  Postive Sequence/1(posSeq) -> If Action Subsystem/1(V)
  Merge/1 -> Freq/1
  If Action Subsystem1/1(Out1) -> Merge/2
  If Action Subsystem/1(Freq) -> Merge/1
  Constant/1 -> Discrete-Time Integrator/1
  abc/1 -> Postive Sequence/1(abc)
  Discrete-Time Integrator/1 -> If/1, If Action Subsystem/2(Time)
  If/2 -> If Action Subsystem1/Action
  If/1 -> If Action Subsystem/Action

== system MicrogridControl/Solar/Solar Plant Integrated/Detailed/PV Plant & Controller/Controller ==
  Qref : Inport
  ipv (A) : Inport  Port=2
  vdc (V) : Inport  Port=3
  Vabc : Inport  Port=4
  Iabc : Inport  Port=5
  Pref : Inport  Port=6
  Mode : Inport  Port=7
  If : If
  MPPT : Subsystem  TreatAsAtomicUnit=on
  Merge : Merge
  Power Reference : Subsystem  TreatAsAtomicUnit=on
  vabcRef (pu) : Outport
  wires:
  ipv (A)/1 -> MPPT/2(ipv (A))
  vdc (V)/1 -> MPPT/3(vdc (V))
  Qref/1 -> MPPT/1(Qref), Power Reference/4(QRef)
  Iabc/1 -> Power Reference/1(Iabc), MPPT/5(Iabc)
  Pref/1 -> Power Reference/3(PRef)
  Vabc/1 -> Power Reference/2(Vabc), MPPT/4(Vabc)
  If/1 -> MPPT/Action
  If/2 -> Power Reference/Action
  MPPT/1(mabc) -> Merge/1
  Power Reference/1(mabc) -> Merge/2
  Merge/1 -> vabcRef (pu)/1
  Mode/1 -> If/1

== system MicrogridControl/Solar/Solar Plant Integrated/Detailed/PV Plant & Controller/PV Plant ==
  mabc : Inport
  Converter : Subsystem  InitFcn=%solar.mask.restoreConverterLink(gcb);  Variant=on  VariantControlMode=label  LabelModeActiveChoice=Average  mask{converterFidelity=Average, fSw=fSw}
      mask prompts: converterFidelity "Converter Fidelity"; fSw "Switching Frequency (kHz)"
      settings: PreSaveFcn=%solar.mask.restoreConverterLink  CloseFcn=%solar.mask.restoreConverterLink
      mask TypeOptions converterFidelity: Average | Switching
      mask Callback converterFidelity: component.mask.converterFidelity(gcb);
      mask DialogControl editSwitch Prompt: Edit converter parameters
      mask DialogControl editSwitch Callback:
      | converterFidelity = get_param(gcb,'converterFidelity');
      | blockPath = [gcb,'/',converterFidelity,'/','Converter'];
      | component.mask.openBlock(blockPath);
  Current Sensor : fl_lib/Electrical/Electrical Sensors/Current Sensor
  DC- Capacitor : fl_lib/Electrical/Electrical Elements/Capacitor  c=capDC F  r=1e-6 Ohm  g=0 1/Ohm  i_specify=off  i_priority=None  i=0 A  i_nominal_specify=off  i_nominal_value=1  i_nominal_unit=A  v_specify=off  v_priority=None  v=6560*.5 V  v_nominal_specify=off  v_nominal_value=1  v_nominal_unit=V  vc_specify=on  vc_priority=None  vc=ceil(Vac*sqrt(2)*1.2) V  vc_nominal_specify=off  vc_nominal_value=1  vc_nominal_unit=V
  ERef1 : fl_lib/Electrical/Electrical Elements/Electrical Reference
  PS-Simulink Converter : nesl_utility/PS-Simulink Converter  PhysicalDomain=network_engine_domain  SubClassName=ps_output  LeftPortType=input  RightPortType=output  PseudoPeriodic=off  Frequencies=[]  VectorFormat=inherit  Unit=inherit  AffineConversion=off
  PS-Simulink Converter1 : nesl_utility/PS-Simulink Converter  PhysicalDomain=network_engine_domain  SubClassName=ps_output  LeftPortType=input  RightPortType=output  PseudoPeriodic=off  Frequencies=[]  VectorFormat=inherit  Unit=inherit  AffineConversion=off
  PV Array : ee_lib/Sources/Solar Cell  PartSpecification="{\"CollectionId\":\"SimscapeElectrical\",\"DatasetId\":\"Tata_Power_Solar|TP300|simscape.electrical.solarCell\",\"DisplayName\":\"Tata_Power_Solar:TP300\"}"  prm=ee.enum.sources.solar_cell_prm.fiveParameter  Isc=8.71 % Datasheet derived A  Voc=0.62223 % Datasheet derived V  Is=1.08146075786774e-06 % Datasheet derived A  Is2=5.42602984007438e-09 % Datasheet derived A  Iph=8.71000410148422 % Datasheet derived A  Ir0=1000 % Datasheet derived W/m^2  ec=1.52301308864556 % Datasheet derived  N2=1.87068753668451 % Datasheet derived  Rs=0.000339119125335165 % Datasheet derived Ohm  Rp=655.536158839936 % Datasheet derived Ohm  N_series=72*nSeries% Datasheet derived  N_parallel=1*nParallel % Datasheet derived  TIPH1=0.000579985599628516 % Datasheet derived 1/K  EG=1.12 % Datasheet derived eV  TXIS1=3.78147935095899 % Datasheet derived  TXIS2=12.1162776751811 % Datasheet derived  TRS1=0.141899818875295 % Datasheet derived  TRP1=0 % Parameter not set  Tmeas=25 % Datasheet derived degC  TFIXED=25 % Datasheet derived degC  thermal_mass=100 % Parameter not set J/K  initial_temperature=25 degC
      settings: AttributesFormatString=Tata_Power_Solar:TP300
  Voltage Sensor : fl_lib/Electrical/Electrical Sensors/Voltage Sensor
  ABC : PMIOPort  Side=Right
  Ir : PMIOPort  Port=2  Side=Left
  I : Outport
  V : Outport  Port=2
  wires:
  PS-Simulink Converter/1 -> I/1
  PS-Simulink Converter1/1 -> V/1
  mabc/1 -> Converter/1(mabc)
  connections:
  PV Array/LConn2 -- Current Sensor/LConn1
  ABC/RConn1 -- Converter/RConn1
  Ir/RConn1 -- PV Array/LConn1
  PS-Simulink Converter/LConn1 -- Current Sensor/RConn1
  PS-Simulink Converter1/LConn1 -- Voltage Sensor/RConn1
  DC- Capacitor/LConn1 -- Converter/LConn1 -- Current Sensor/RConn2 -- Voltage Sensor/LConn1
  DC- Capacitor/RConn1 -- Converter/LConn2 -- ERef1/LConn1 -- PV Array/RConn1 -- Voltage Sensor/RConn2

== system MicrogridControl/Solar/Solar Plant Integrated/Detailed/PV Plant & Controller/Sensor Dynamics ==
  Iin : Inport
  Vin : Inport  Port=2
  Current Measurement : Subsystem
  Product : Product
  Scope : Scope
      settings: ActiveDisplayYMinimum=-1.17977100562E+6  ActiveDisplayYMaximum=5.50264896669E+6  DataLoggingVariableName=ScopeData5
  Voltage Measurement : Subsystem
  I : Outport
  V : Outport  Port=2
  wires:
  Current Measurement/1(V) -> Product/2, I/1
  Iin/1 -> Current Measurement/1(u)
  Vin/1 -> Voltage Measurement/1(u)
  Voltage Measurement/1(I) -> Product/1, V/1
  Product/1 -> Scope/1

== system MicrogridControl/Solar/Solar Plant Integrated1/Detailed/PV Plant & Controller/Controller ==
  Qref : Inport
  ipv (A) : Inport  Port=2
  vdc (V) : Inport  Port=3
  Vabc : Inport  Port=4
  Iabc : Inport  Port=5
  Pref : Inport  Port=6
  Mode : Inport  Port=7
  If : If
  MPPT : Subsystem  TreatAsAtomicUnit=on
  Merge : Merge
  Power Reference : Subsystem  TreatAsAtomicUnit=on
  vabcRef (pu) : Outport
  wires:
  ipv (A)/1 -> MPPT/2(ipv (A))
  vdc (V)/1 -> MPPT/3(vdc (V))
  Qref/1 -> MPPT/1(Qref), Power Reference/4(QRef)
  Iabc/1 -> Power Reference/1(Iabc), MPPT/5(Iabc)
  Pref/1 -> Power Reference/3(PRef)
  Vabc/1 -> Power Reference/2(Vabc), MPPT/4(Vabc)
  If/1 -> MPPT/Action
  If/2 -> Power Reference/Action
  MPPT/1(mabc) -> Merge/1
  Power Reference/1(mabc) -> Merge/2
  Merge/1 -> vabcRef (pu)/1
  Mode/1 -> If/1
